simulink model "Scenario_MinimumExample_TwithoutTrafficLights_tol_fixed"  (R2021a)
settings: Solver=VariableStepAuto  StartTime=0.0  StopTime=50  RelTol=1e-3
model workspace (MAT data in the model file):
  Kz_dif : Simulink.Parameter (value not decoded)
  Kz_il : Simulink.Parameter (value not decoded)
  Kz_ir : Simulink.Parameter (value not decoded)
  Kz_is : Simulink.Parameter (value not decoded)
  Kz_long : Simulink.Parameter (value not decoded)
  Kz_pre : Simulink.Parameter (value not decoded)
  L_dif : Simulink.Parameter (value not decoded)
  L_il : Simulink.Parameter (value not decoded)
  L_ir : Simulink.Parameter (value not decoded)
  L_is : Simulink.Parameter (value not decoded)
  L_long : Simulink.Parameter (value not decoded)
  L_pre : Simulink.Parameter (value not decoded)
  Lc : Simulink.Parameter (value not decoded)
  Rk : Simulink.Parameter (value not decoded)
  Tz_dif : Simulink.Parameter (value not decoded)
  Tz_il : Simulink.Parameter (value not decoded)
  Tz_ir : Simulink.Parameter (value not decoded)
  Tz_is : Simulink.Parameter (value not decoded)
  Tz_long : Simulink.Parameter (value not decoded)
  Tz_pre : Simulink.Parameter (value not decoded)
  ds : Simulink.Parameter (value not decoded)
  dt : Simulink.Parameter (value not decoded)
  v : Simulink.Parameter (value not decoded)
symbols that are objects in the model workspace (value not decoded): Kz_dif, Kz_il, Kz_ir, Kz_is, Kz_long, Kz_pre, Rk, Tz_dif, Tz_il, Tz_ir, Tz_is, Tz_long, Tz_pre
libraries: StreetLanesLibrary x72, EdgesLibrary x64, MeasuringLibrary x34, SourcesAndSinksLibrary x11
(part 3 of 3)

== stateflow chart Scenario_MinimumExample_TwithoutTrafficLights_tol_fixed/Plus-Controller ==
  state CompleteController
    state timecounter [parallel]
      settings: executionOrder=1
    state actualController [parallel]
      settings: executionOrder=2
      (history)
      note: ?
      state Group__Crs_Brs
      state Group__Cl_Bl
      state Group__Ars_Drs
      state Group__Al_Dl
      note: check
          | Crs straight
          | crossings
      note: check
          | Cl
          | crossings
      note: check
          | Ars straight
          | crossings
      note: check
          | Al
          | crossings
      note: check
          | Crs right
          | crossings
      note: check
          | Bl
          | crossings
      note: check
          | Ars right
          | crossings
      note: check
          | Dl
          | crossings
      note: check
          | Brs straight
          | crossings
      note: check
          | Drs straight
          | crossings
      note: check
          | Brs right
          | crossings
      note: check
          | Drs right
          | crossings
      Group__Al_Dl -> Group__Crs_Brs [order 1] : [time >= green_duration_l]
          | {enAl = 0; enDl = 0; time = 0;}
      Group__Ars_Drs -> Group__Al_Dl [order 1] : [time >=green_duration_sr]
          | {enAs = 0; enAr = 0; enDs = 0; enDr = 0; time = 0;}
      Group__Cl_Bl -> Group__Ars_Drs [order 1] : [time >= green_duration_l]
          | {enCl = 0; enBl = 0; time = 0;}
      Group__Crs_Brs -> Group__Cl_Bl [order 1] : [time >= green_duration_sr]
          | {enCs = 0; enCr = 0; enBs = 0;
          | enBr = 0; time = 0;}
      (default) -> Group__Crs_Brs : {enAl = 0; enAs = 0; enAr = 0;
          | enBl = 0; enBs = 0; enBr = 0;
          | enCl = 0; enCs = 0; enCr = 0;
          | enDl = 0; enDs = 0; enDr = 0;}
      Group__Crs_Brs -> (junction 51) [order 2]
      (junction 109) -> Group__Crs_Brs
      Group__Cl_Bl -> (junction 117) [order 2]
      (junction 126) -> Group__Cl_Bl
      Group__Ars_Drs -> (junction 134) [order 2]
      (junction 131) -> Group__Ars_Drs
      Group__Al_Dl -> (junction 151) [order 2]
      (junction 160) -> Group__Al_Dl
      (junction 117) -> (junction 116) [order 2] : {enCl = 0;}
      (junction 51) -> (junction 59) [order 1] : [(Dl_Co<=tol && Drs_Ao<=tol ...
          | && Drs_Bo<=tol && Bl_Do<=tol ...
          | && Al_Bo<=tol && Ars_Do<=tol)]
          | {enCs = 1;}
      (junction 117) -> (junction 116) [order 1] : [Dl_Co<=tol && Drs_Ao<=tol && ....
          | Brs_Co<=tol && Al_Bo<=tol && ...
          | Ars_Do<=tol && Brs_Ao]{enCl = 1;}
      (junction 51) -> (junction 59) [order 2] : {enCs = 0;}
      (junction 134) -> (junction 133) [order 1] : [Cl_Ao<=tol && Crs_Bo<=tol && ...
          | Crs_Do<=tol && Dl_Co<=tol && ...
          | Bl_Do<=tol && Brs_Co<=tol]
          | {enAs = 1;}
      (junction 151) -> (junction 150) [order 1] : [(Cl_Ao<=tol && Crs_Bo<=tol ...
          | && Drs_Ao<=tol && Bl_Do<=tol ...
          | && Brs_Co<=tol && Drs_Bo)]{enAl = 1;}
      (junction 134) -> (junction 133) [order 2] : {enAs = 0;}
      (junction 151) -> (junction 150) [order 2] : {enAl = 0;}
      (junction 59) -> (junction 104) [order 1] : [(Ars_Do<=tol && Bl_Do<=tol)]
          | {enCr = 1;}
      (junction 116) -> (junction 126) [order 1] : [(Al_Bo<=tol && Ars_Do<=tol && ...
          | Crs_Bo<=tol && Dl_Co<=tol && ...
          | Drs_Ao<=tol && Crs_Do)]{enBl = 1;}
      (junction 59) -> (junction 104) [order 2] : {enCr = 0;}
      (junction 116) -> (junction 126) [order 2] : {enBl = 0;}
      (junction 133) -> (junction 143) [order 1] : [(Brs_Co<=tol && Dl_Co<=tol)]
          | {enAr = 1;}
      (junction 150) -> (junction 160) [order 1] : [(Bl_Do<=tol && Brs_Co<=tol ...
          | && Ars_Do<=tol && Cl_Ao<=tol ...
          | && Crs_Bo<=tol && Ars_Co)]{enDl = 1;}
      (junction 133) -> (junction 143) [order 2] : {enAr = 0;}
      (junction 150) -> (junction 160) [order 2] : {enDl = 0;}
      (junction 104) -> (junction 105) [order 1] : [(Al_Bo<=tol && Ars_Do<=tol ...
          | && Ars_Co<=tol && Cl_Ao<=tol ...
          | && Dl_Co<=tol && Drs_Ao<=tol)]
          | {enBs = 1;}
      (junction 104) -> (junction 105) [order 2] : {enBs = 0;}
      (junction 143) -> (junction 141) [order 1] : [(Bl_Do<=tol && Brs_Co<=tol ...
          | && Brs_Ao<=tol && Al_Bo<=tol ...
          | && Cl_Ao<=tol && Crs_Bo<=tol)]
          | {enDs = 1;}
      (junction 143) -> (junction 141) [order 2] : {enDs=0;}
      (junction 105) -> (junction 109) [order 1] : [Drs_Ao<=tol && Cl_Ao<=tol]
          | {enBr = 1;}
      (junction 105) -> (junction 109) [order 2] : {enBr = 0;}
      (junction 141) -> (junction 131) [order 1] : [(Crs_Bo<=tol && Al_Bo<=tol)]
          | {enDr = 1;}
      (junction 141) -> (junction 131) [order 2] : {enDr = 0;}
    timecounter -> timecounter : [after(1,sec)]{time=time+1;}
  (default) -> CompleteController : {enAl = 0; enAs = 0; enAr = 0;
      | enBl = 0; enBs = 0; enBr = 0;
      | enCl = 0; enCs = 0; enCr = 0;
      | enDl = 0; enDs = 0; enDr = 0;
      | time = 0;}
  data: Bl input; Brs input; Al input; Ars input; Cl input; Crs input; Dl input; Drs input; Al_Bo input; Ars_Do input; Ars_Co input; Bl_Do input; Brs_Co input; Brs_Ao input; Cl_Ao input; Crs_Bo input; Crs_Do input; Dl_Co input; Drs_Ao input; Drs_Bo input; enAl output =0; enAs output =0; enAr output =0; enBl output =0; enBs output =0; enBr output =0; enCl output =0; enCs output =0; enCr output =0; enDl output =0; enDs output =0; enDr output =0; green_duration_sr parameter; green_duration_l parameter; tol parameter; time output
